simulink model "base_case_anderson_v2"  (R2015b)
settings: Solver=FixedStepAuto  StartTime=0.0  StopTime=45  FixedStep=Ts  RelTol=1e-3
undefined symbols (not defined in the file): Cbase, Lbase, Ts, Xbase
libraries: powerlib x127, powerlib_meascontrol x19, sps_avr x3
(part 2 of 2)

== system base_case_anderson_v2/Line 7-8/B//1 ==
  Ground : powerlib/Elements/Ground  LConnTagsString=a
  R2-1 : powerlib/Elements/Series RLC Branch  LConnTagsString=__new0  RConnTagsString=__new0  BranchType=C  Resistance=1  Inductance=1e-3  SetiL0=off  InitialCurrent=0  Capacitance=Cbase*0.0745  Setx0=off  InitialVoltage=0  Measurements=None
  R2-2 : powerlib/Elements/Series RLC Branch  LConnTagsString=__new0  RConnTagsString=__new0  BranchType=C  Resistance=1  Inductance=1e-3  SetiL0=off  InitialCurrent=0  Capacitance=Cbase*0.0745  Setx0=off  InitialVoltage=0  Measurements=None
  R2-3 : powerlib/Elements/Series RLC Branch  LConnTagsString=__new0  RConnTagsString=__new0  BranchType=C  Resistance=1  Inductance=1e-3  SetiL0=off  InitialCurrent=0  Capacitance=Cbase*0.0745  Setx0=off  InitialVoltage=0  Measurements=None
  Conn1 : PMIOPort  Port=1  Side=Right
  Conn2 : PMIOPort  Port=2  Side=Right
  Conn3 : PMIOPort  Port=3  Side=Right
  connections:
  R2-3/LConn1 -- Conn1/RConn1
  R2-2/RConn1 -- R2-3/RConn1 -- Ground/LConn1 -- R2-1/RConn1
  R2-2/LConn1 -- Conn3/RConn1
  R2-1/LConn1 -- Conn2/RConn1

== system base_case_anderson_v2/Line 7-8/B//2 ==
  Ground : powerlib/Elements/Ground  LConnTagsString=a
  R2-1 : powerlib/Elements/Series RLC Branch  LConnTagsString=__new0  RConnTagsString=__new0  BranchType=C  Resistance=1  Inductance=1e-3  SetiL0=off  InitialCurrent=0  Capacitance=Cbase*0.0745  Setx0=off  InitialVoltage=0  Measurements=None
  R2-2 : powerlib/Elements/Series RLC Branch  LConnTagsString=__new0  RConnTagsString=__new0  BranchType=C  Resistance=1  Inductance=1e-3  SetiL0=off  InitialCurrent=0  Capacitance=Cbase*0.0745  Setx0=off  InitialVoltage=0  Measurements=None
  R2-3 : powerlib/Elements/Series RLC Branch  LConnTagsString=__new0  RConnTagsString=__new0  BranchType=C  Resistance=1  Inductance=1e-3  SetiL0=off  InitialCurrent=0  Capacitance=Cbase*0.0745  Setx0=off  InitialVoltage=0  Measurements=None
  Conn1 : PMIOPort  Port=1  Side=Right
  Conn2 : PMIOPort  Port=2  Side=Right
  Conn3 : PMIOPort  Port=3  Side=Right
  connections:
  R2-1/LConn1 -- Conn2/RConn1
  R2-2/LConn1 -- Conn3/RConn1
  Ground/LConn1 -- R2-2/RConn1 -- R2-1/RConn1 -- R2-3/RConn1
  R2-3/LConn1 -- Conn1/RConn1

== system base_case_anderson_v2/Line 8-9/B//1 ==
  Ground : powerlib/Elements/Ground  LConnTagsString=a
  R2-1 : powerlib/Elements/Series RLC Branch  LConnTagsString=__new0  RConnTagsString=__new0  BranchType=C  Resistance=1  Inductance=1e-3  SetiL0=off  InitialCurrent=0  Capacitance=Cbase*0.1045  Setx0=off  InitialVoltage=0  Measurements=None
  R2-2 : powerlib/Elements/Series RLC Branch  LConnTagsString=__new0  RConnTagsString=__new0  BranchType=C  Resistance=1  Inductance=1e-3  SetiL0=off  InitialCurrent=0  Capacitance=Cbase*0.1045  Setx0=off  InitialVoltage=0  Measurements=None
  R2-3 : powerlib/Elements/Series RLC Branch  LConnTagsString=__new0  RConnTagsString=__new0  BranchType=C  Resistance=1  Inductance=1e-3  SetiL0=off  InitialCurrent=0  Capacitance=Cbase*0.1045  Setx0=off  InitialVoltage=0  Measurements=None
  Conn1 : PMIOPort  Port=1  Side=Right
  Conn2 : PMIOPort  Port=2  Side=Right
  Conn3 : PMIOPort  Port=3  Side=Right
  connections:
  R2-1/LConn1 -- Conn2/RConn1
  R2-2/LConn1 -- Conn3/RConn1
  R2-3/RConn1 -- Ground/LConn1 -- R2-2/RConn1 -- R2-1/RConn1
  R2-3/LConn1 -- Conn1/RConn1

== system base_case_anderson_v2/Line 8-9/B//2 ==
  Ground : powerlib/Elements/Ground  LConnTagsString=a
  R2-1 : powerlib/Elements/Series RLC Branch  LConnTagsString=__new0  RConnTagsString=__new0  BranchType=C  Resistance=1  Inductance=1e-3  SetiL0=off  InitialCurrent=0  Capacitance=Cbase*0.1045  Setx0=off  InitialVoltage=0  Measurements=None
  R2-2 : powerlib/Elements/Series RLC Branch  LConnTagsString=__new0  RConnTagsString=__new0  BranchType=C  Resistance=1  Inductance=1e-3  SetiL0=off  InitialCurrent=0  Capacitance=Cbase*0.1045  Setx0=off  InitialVoltage=0  Measurements=None
  R2-3 : powerlib/Elements/Series RLC Branch  LConnTagsString=__new0  RConnTagsString=__new0  BranchType=C  Resistance=1  Inductance=1e-3  SetiL0=off  InitialCurrent=0  Capacitance=Cbase*0.1045  Setx0=off  InitialVoltage=0  Measurements=None
  Conn1 : PMIOPort  Port=1  Side=Right
  Conn2 : PMIOPort  Port=2  Side=Right
  Conn3 : PMIOPort  Port=3  Side=Right
  connections:
  R2-3/LConn1 -- Conn1/RConn1
  R2-2/RConn1 -- R2-3/RConn1 -- R2-1/RConn1 -- Ground/LConn1
  R2-2/LConn1 -- Conn3/RConn1
  R2-1/LConn1 -- Conn2/RConn1

== system base_case_anderson_v2/Line 9-6/B//1 ==
  Ground : powerlib/Elements/Ground  LConnTagsString=a
  R2-1 : powerlib/Elements/Series RLC Branch  LConnTagsString=__new0  RConnTagsString=__new0  BranchType=C  Resistance=1  Inductance=1e-3  SetiL0=off  InitialCurrent=0  Capacitance=Cbase*0.179  Setx0=off  InitialVoltage=0  Measurements=None
  R2-2 : powerlib/Elements/Series RLC Branch  LConnTagsString=__new0  RConnTagsString=__new0  BranchType=C  Resistance=1  Inductance=1e-3  SetiL0=off  InitialCurrent=0  Capacitance=Cbase*0.179  Setx0=off  InitialVoltage=0  Measurements=None
  R2-3 : powerlib/Elements/Series RLC Branch  LConnTagsString=__new0  RConnTagsString=__new0  BranchType=C  Resistance=1  Inductance=1e-3  SetiL0=off  InitialCurrent=0  Capacitance=Cbase*0.179  Setx0=off  InitialVoltage=0  Measurements=None
  Conn1 : PMIOPort  Port=1  Side=Right
  Conn2 : PMIOPort  Port=2  Side=Right
  Conn3 : PMIOPort  Port=3  Side=Right
  connections:
  R2-1/LConn1 -- Conn2/RConn1
  R2-2/LConn1 -- Conn3/RConn1
  R2-2/RConn1 -- Ground/LConn1 -- R2-3/RConn1 -- R2-1/RConn1
  R2-3/LConn1 -- Conn1/RConn1

== system base_case_anderson_v2/Line 9-6/B//2 ==
  Ground : powerlib/Elements/Ground  LConnTagsString=a
  R2-1 : powerlib/Elements/Series RLC Branch  LConnTagsString=__new0  RConnTagsString=__new0  BranchType=C  Resistance=1  Inductance=1e-3  SetiL0=off  InitialCurrent=0  Capacitance=Cbase*0.179  Setx0=off  InitialVoltage=0  Measurements=None
  R2-2 : powerlib/Elements/Series RLC Branch  LConnTagsString=__new0  RConnTagsString=__new0  BranchType=C  Resistance=1  Inductance=1e-3  SetiL0=off  InitialCurrent=0  Capacitance=Cbase*0.179  Setx0=off  InitialVoltage=0  Measurements=None
  R2-3 : powerlib/Elements/Series RLC Branch  LConnTagsString=__new0  RConnTagsString=__new0  BranchType=C  Resistance=1  Inductance=1e-3  SetiL0=off  InitialCurrent=0  Capacitance=Cbase*0.179  Setx0=off  InitialVoltage=0  Measurements=None
  Conn1 : PMIOPort  Port=1  Side=Right
  Conn2 : PMIOPort  Port=2  Side=Right
  Conn3 : PMIOPort  Port=3  Side=Right
  connections:
  R2-3/LConn1 -- Conn1/RConn1
  R2-3/RConn1 -- R2-2/RConn1 -- R2-1/RConn1 -- Ground/LConn1
  R2-2/LConn1 -- Conn3/RConn1
  R2-1/LConn1 -- Conn2/RConn1
